simulink model "test"  (R2023b)
settings: Solver=VariableStepAuto  StartTime=0.0  StopTime=10.0  RelTol=1e-3
settings Model: Creator=86186  LastModifiedBy=86186

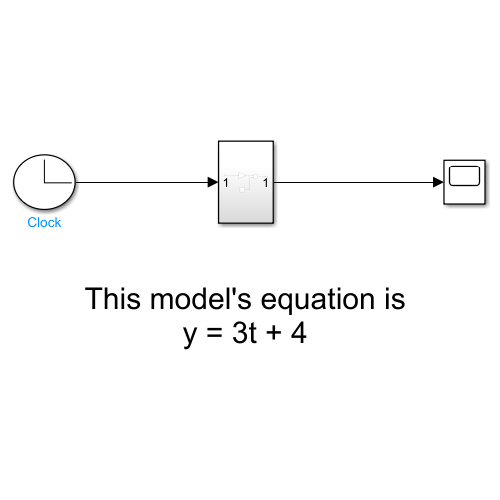
[thumbnail: Simulink's stored preview of the top-level diagram]
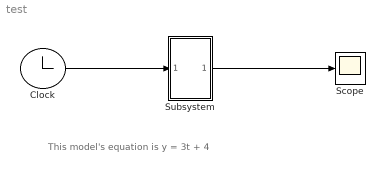
== system test ==
  note: This model's equation is
      | y = 3t + 4
  Clock : Clock
  Scope : Scope
  Subsystem : Subsystem
  wires:
  Clock/1 -> Subsystem/1(In1)
  Subsystem/1(Out1) -> Scope/1

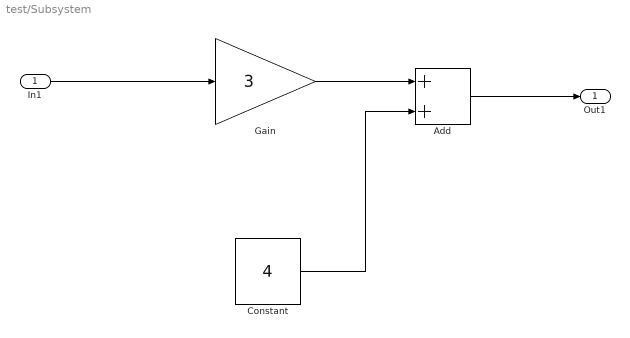
== system test/Subsystem ==
  In1 : Inport
  Add : Sum
  Constant : Constant  Value=4
  Gain : Gain  Gain=3
  Out1 : Outport
  wires:
  Add/1 -> Out1/1
  Gain/1 -> Add/1
  Constant/1 -> Add/2
  In1/1 -> Gain/1
